simulink subsystem "PieroHW"  (R2024b)
settings: Solver=VariableStepAuto  StartTime=0.0  StopTime=10.0  RelTol=1e-3
libraries: simulink x1
settings Model: Creator=Chenfu  LastModifiedBy=Chenfu

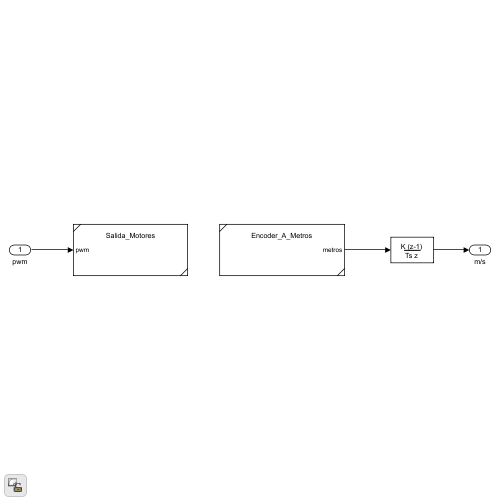
[thumbnail: Simulink's stored preview of the top-level diagram]
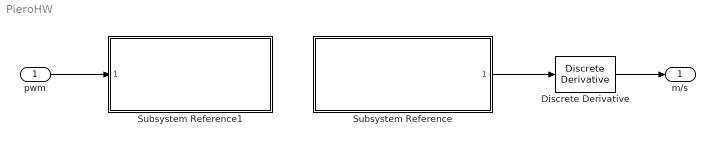
== system PieroHW ==
  pwm : Inport
  Discrete Derivative : simulink/Discrete/Discrete Derivative  gainval=1.0  ICPrevScaledInput=0.0  OutMin=[]  OutMax=[]  OutDataTypeStr=double  OutputDataTypeScalingMode=double  OutDataType=fixdt(1, 16)  OutScaling=2^-10  DoSatur=off
  Subsystem Reference : Subsystem  ReferencedSubsystem=Encoder_A_Metros
  Subsystem Reference1 : Subsystem  ReferencedSubsystem=Salida_Motores
  m/s : Outport
  wires:
  pwm/1 -> Subsystem Reference1/1
  Subsystem Reference/1 -> Discrete Derivative/1
  Discrete Derivative/1 -> m/s/1
